simulink model "readMagnetometer"  (R2019a)
settings: Solver=FixedStepAuto  StartTime=0.0  StopTime=inf  RelTol=1e-3  EnableMultiTasking=on
libraries: raspberrypilib x6, simulink x1
settings Model: SimulationMode=external  Creator=florian  LastModifiedBy=florian
settings SolverCC: PositivePriorityOrder=on
settings OptimizationCC: EnhancedBackFolding=on  PassReuseOutputArgsAs=Individual arguments  MaxStackSize=64  OptimizeBlockOrder=speed  DifferentSizesBufferReuse=on  OptimizationCustomize=off
settings DebuggingCC: ParameterTunabilityLossMsg=error
settings HardwareCC: ProdBitPerPointer=32  ProdBitPerSizeT=32  ProdBitPerPtrDiffT=32  ProdLargestAtomicInteger=Long  ProdLargestAtomicFloat=Double  ProdWordSize=32  ProdLongLongMode=on  ProdHWDeviceType=ARM Compatible->ARM Cortex
settings SFSimCC: MATLABDynamicMemAlloc=off
settings RTWCC: SystemTargetFile=ert.tlc  HardwareBoard=Raspberry Pi  TLCOptions="-aInlineSetEventsForThisBaseRateFcn=TLC_FALSE -aSuppressMultiTaskScheduler=TLC_FALSE  -aRateBasedStepFcn=0"  TemplateMakefile=ert_default_tmf  GenerateReport=on  Toolchain=GNU GCC Raspberry Pi  BuildConfiguration=Faster Runs  IncludeHyperlinkInReport=on  LaunchReport=on  GenerateTraceInfo=on  GenerateTraceReport=on  GenerateTraceReportSl=on  GenerateTraceReportSf=on  GenerateTraceReportEml=on
settings CodeAppCC: ForceParamTrailComments=on  IgnoreCustomStorageClasses=off  OperatorAnnotations=on  SimulinkDataObjDesc=on  SFDataObjDesc=on  InsertBlockDesc=on
settings ERTTargetCC: SupportContinuousTime=on  SupportVariableSizeSignals=on

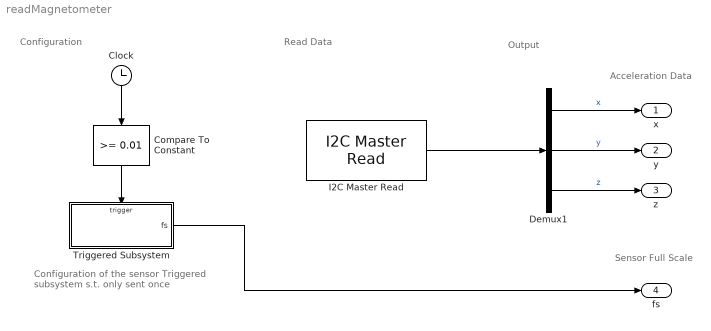
== system readMagnetometer ==
  note: Configuration
  note: Configuration of the sensor
      | Triggered subsystem s.t. only sent once
  note: Read Data
  note: Output
  note: Acceleration Data
  note: Sensor Full Scale
  Clock : Clock
  Compare To Constant : simulink/Logic and Bit Operations/Compare To Constant  relop=>=  const=0.01  OutDataTypeStr=boolean
  Demux1 : Demux  Outputs=3
  I2C Master Read : raspberrypilib/I2C Master Read  BoardProperty=Pi 3 Model B+  Mode=Master  SlaveAddress=30  SlaveByteOrder=LittleEndian  Direction=Receiver  RegisterAddressMode=on  RegisterAddress=40  SlaveDataType=int16  DataLength=3  NoAck=off  RepeatedStart=off  OutputStatus=off  SampleTime=0.0006
      settings: SourceProductName=Simulink Support Package for Raspberry Pi Hardware  SourceProductBaseCode=RASPPI
  Triggered Subsystem : Subsystem  TreatAsAtomicUnit=on
  x : Outport
  y : Outport  Port=2
  z : Outport  Port=3
  fs : Outport  Port=4
  wires:
  I2C Master Read/1 -> Demux1/1
  Demux1/1 -> x/1  "x"
  Demux1/2 -> y/1  "y"
  Demux1/3 -> z/1  "z"
  Compare To Constant/1 -> Triggered Subsystem/Trigger
  Clock/1 -> Compare To Constant/1
  Triggered Subsystem/1(fs) -> fs/1

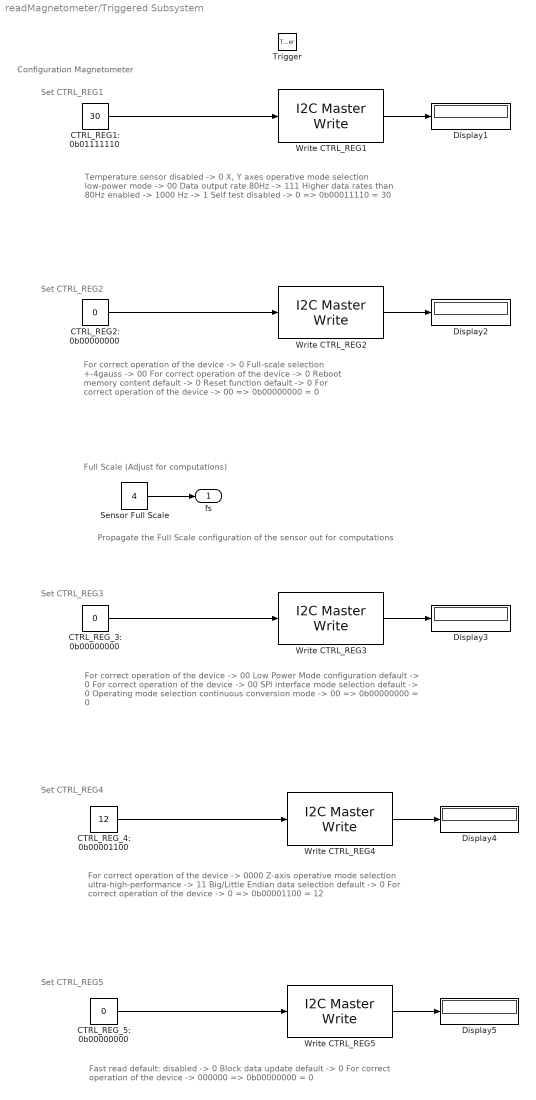
== system readMagnetometer/Triggered Subsystem ==
  note: Set CTRL_REG1
  note: Fast read							default: disabled		-> 0
      | Block data update					default				-> 0
      | For correct operation of the device							-> 000000
      | 									=> 0b00000000 = 0
  note: For correct operation of the device								-> 0000
      | Z-axis operative mode selection		ultra-high-performance	-> 11
      | Big/Little Endian data selection			default					-> 0
      | For correct operation of the device								-> 0
      | 									=> 0b00001100 = 12
  note: For correct operation of the device									-> 00
      | Low Power Mode configuration			default						-> 0
      | For correct operation of the device									-> 00
      | SPI interface mode selection			default						-> 0
      | Operating mode selection				continuous conversion mode 	-> 00
      | 									=> 0b00000000 = 0
  note: For correct operation of the device -> 0
      | Full-scale selection +-4gauss -> 00
      | For correct operation of the device -> 0
      | Reboot memory content default -> 0
      | Reset function default -> 0
      | For correct operation of the device -> 00
      | => 0b00000000 = 0
  note: Temperature sensor					disabled					-> 0
      | X, Y axes operative mode selection		low-power mode			-> 00
      | Data output rate						80Hz					-> 111
      | Higher data rates than 80Hz			enabled -> 1000 Hz		-> 1
      | Self test 								disabled					-> 0
      | 									=> 0b00011110 = 30
  note: Configuration Magnetometer
  note: Full Scale (Adjust for computations)
  note: Propagate the Full Scale configuration of the sensor out for computations
  note: Set CTRL_REG2
  note: Set CTRL_REG3
  note: Set CTRL_REG4
  note: Set CTRL_REG5
  Trigger : TriggerPort  VariantControl=Variant
  CTRL_REG1: 0b01111110 : Constant  Value=30  OutDataTypeStr=uint8
  CTRL_REG2: 0b00000000 : Constant  Value=0  OutDataTypeStr=uint8
  CTRL_REG_3: 0b00000000 : Constant  Value=0  OutDataTypeStr=uint8
  CTRL_REG_4: 0b00001100 : Constant  Value=12  OutDataTypeStr=uint8
  CTRL_REG_5: 0b00000000 : Constant  Value=0  OutDataTypeStr=uint8
  Display{1..5} (5 alike) : Display
  Sensor Full Scale : Constant  Value=4
  Write CTRL_REG1 : raspberrypilib/I2C Master Write  Priority=0  BoardProperty=Pi 3 Model B+  Mode=Master  SlaveAddress=30  SlaveByteOrder=LittleEndian  Direction=Transmitter  RegisterAddressMode=on  RegisterAddress=32  SlaveDataType=uint8  DataLength=1  NoAck=off  RepeatedStart=off  OutputStatus=on
      settings: SourceProductName=Simulink Support Package for Raspberry Pi Hardware  SourceProductBaseCode=RASPPI
  Write CTRL_REG2 : raspberrypilib/I2C Master Write  Priority=0  BoardProperty=Pi 3 Model B+  Mode=Master  SlaveAddress=30  SlaveByteOrder=LittleEndian  Direction=Transmitter  RegisterAddressMode=on  RegisterAddress=33  SlaveDataType=uint8  DataLength=1  NoAck=off  RepeatedStart=off  OutputStatus=on
      settings: SourceProductName=Simulink Support Package for Raspberry Pi Hardware  SourceProductBaseCode=RASPPI
  Write CTRL_REG3 : raspberrypilib/I2C Master Write  Priority=0  BoardProperty=Pi 3 Model B+  Mode=Master  SlaveAddress=30  SlaveByteOrder=LittleEndian  Direction=Transmitter  RegisterAddressMode=on  RegisterAddress=34  SlaveDataType=uint8  DataLength=1  NoAck=off  RepeatedStart=off  OutputStatus=on
      settings: SourceProductName=Simulink Support Package for Raspberry Pi Hardware  SourceProductBaseCode=RASPPI
  Write CTRL_REG4 : raspberrypilib/I2C Master Write  Priority=0  BoardProperty=Pi 3 Model B+  Mode=Master  SlaveAddress=30  SlaveByteOrder=LittleEndian  Direction=Transmitter  RegisterAddressMode=on  RegisterAddress=35  SlaveDataType=uint8  DataLength=1  NoAck=off  RepeatedStart=off  OutputStatus=on
      settings: SourceProductName=Simulink Support Package for Raspberry Pi Hardware  SourceProductBaseCode=RASPPI
  Write CTRL_REG5 : raspberrypilib/I2C Master Write  Priority=0  BoardProperty=Pi 3 Model B+  Mode=Master  SlaveAddress=30  SlaveByteOrder=LittleEndian  Direction=Transmitter  RegisterAddressMode=on  RegisterAddress=36  SlaveDataType=uint8  DataLength=1  NoAck=off  RepeatedStart=off  OutputStatus=on
      settings: SourceProductName=Simulink Support Package for Raspberry Pi Hardware  SourceProductBaseCode=RASPPI
  fs : Outport
  wires:
  Write CTRL_REG3/1 -> Display3/1
  CTRL_REG_4: 0b00001100/1 -> Write CTRL_REG4/1
  CTRL_REG2: 0b00000000/1 -> Write CTRL_REG2/1
  Write CTRL_REG2/1 -> Display2/1
  Write CTRL_REG5/1 -> Display5/1
  Write CTRL_REG4/1 -> Display4/1
  CTRL_REG_5: 0b00000000/1 -> Write CTRL_REG5/1
  Write CTRL_REG1/1 -> Display1/1
  CTRL_REG_3: 0b00000000/1 -> Write CTRL_REG3/1
  CTRL_REG1: 0b01111110/1 -> Write CTRL_REG1/1
  Sensor Full Scale/1 -> fs/1
